simulink model "HT07CombinedPowertrainThermalModelv2IsolatedMotors"  (R2022b)
settings: Solver=VariableStepAuto  StartTime=0.0  StopTime=timeEnd  RelTol=1e-2
values from neighbouring files (symbols this model uses):
  radiator = dualPassRadiatorInit(radiator)    [HT07CombinedPowertrainThermalSetup.m]
  Tamb = 26    [HT07CombinedPowertrainThermalSetup.m]    (also in HT07PowertrainThermalSetup.m = 33; HT07PowertrainThermalSetupExperimental.m)
undefined symbols (not defined in the file or in its folder): AH, convectionArea, DiscIntNeverNeededParam, SOC0, startTempC, tabResis
libraries: fl_lib x165, nesl_utility x43, SimscapeFluids_lib x16, ee_lib x2
(part 2 of 5)

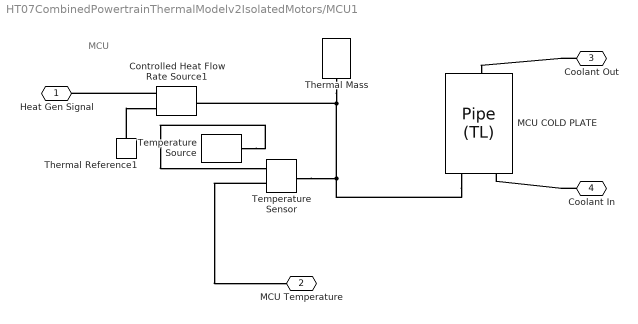
== system HT07CombinedPowertrainThermalModelv2IsolatedMotors/MCU1 ==
  note: MCU
  Controlled Heat Flow Rate Source1 : fl_lib/Thermal/Thermal Sources/Controlled Heat Flow Rate Source
  MCU COLD PLATE : SimscapeFluids_lib/Thermal Liquid/Pipes & Fittings/Pipe (TL)  dynamic_compressibility=simscape.enum.onoff.off  inertia=simscape.enum.onoff.off  num_segments=1  pipe_length=mcuColdPlateLength m  area=mcuColdPlateFlowArea m^2  wall_spec=fluids.thermal_liquid.pipes_fittings.enum.wall_spec.rigid  Dh=mcuColdPlateDiameter m  wall_compliance=1.2e-6 m/MPa  wall_time_constant=0.01 s  elevation_spec=foundation.enum.constant_variable.constant  elevation_gain=0 m  g=9.81 m/s^2  pressure_loss_spec=fluids.thermal_liquid.pipes_fittings.enum.PressureLossSpec.Nominal  local_pressure_loss_spec=fluids.thermal_liquid.pipes_fittings.enum.LocalLossSpec.AggregateLength  length_add=0 m  loss_coefficient=0.1  roughness=tubeRoughness m  Re_friction_TLU=[400, 1000, 1500, 3000, 4000, 6000, 10000, 20000, 40000, 60000, 100000, 100000000]  friction_factor_TLU=[.264, .112, .071, .0417, .0387, .0268, .025, .0232, .0226, .022, .0214, .0214]  shape_factor=64  Re_lam=2000  Re_tur=4000  mdot_nominal=12 kg/min  p_diff_nominal=0.3 bar  mdot_threshold=1e-6 kg/s  heat_transfer_spec=fluids.thermal_liquid.pipes_fittings.enum.HeatTransferSpec.DittusBoelter  mdot_nominal_heat=[.1, 1] kg/s  T_in_nominal=[293.15, 293.15] K  T_out_nominal=[300, 300] K  p_in_nominal_heat=[.101325, .101325] MPa  T_wall_nominal=[303.15, 303.15] K  a_coeff=0.023  b_Re_power=0.8  c_Pr_power=0.4  Nu_lam=3.66  Re_Colburn_TLU=[100, 150, 1000]  Colburn_factor_TLU=[.019, .013, .002]  Re_Nu_TLU=[100, 150, 1000]  Pr_Nu_TLU=[1, 10]  Nu_TLU=[3.72, 4.21; 3.75, 4.44; 4.21, 7.15]  T0_vec=Tamb degC  p0_vec=0.101325 MPa  mdot0=0.1 kg/s
  Temperature Sensor : fl_lib/Thermal/Thermal Sensors/Temperature Sensor
  Temperature Source : fl_lib/Thermal/Thermal Sources/Temperature Source  temperature=0 degC
  Thermal Mass : fl_lib/Thermal/Thermal Elements/Thermal Mass  mass=coldPlateMassMCU kg  sp_heat=cAl J/(K*kg)  num_ports=foundation.enum.numPorts2.one  T_specify=on  T_priority=High  T=Tamb degC  T_nominal_specify=off  T_nominal_unit=K  T_nominal_value=1  Q_specify=off  Q_priority=None  Q=0 W  Q_nominal_specify=off  Q_nominal_unit=W  Q_nominal_value=1
  Thermal Reference1 : fl_lib/Thermal/Thermal Elements/Thermal Reference
  Heat Gen Signal : PMIOPort  Side=Left
  MCU Temperature : PMIOPort  Port=2  Side=Left
  Coolant Out : PMIOPort  Port=3  Side=Right
  Coolant In : PMIOPort  Port=4  Side=Right
  connections:
  Temperature Sensor/RConn2 -- MCU Temperature/RConn1
  MCU COLD PLATE/LConn2 -- Temperature Sensor/LConn1 -- Thermal Mass/LConn1 -- Controlled Heat Flow Rate Source1/LConn1
  Temperature Source/LConn1 -- Temperature Sensor/RConn1
  Thermal Reference1/LConn1 -- Controlled Heat Flow Rate Source1/RConn2
  Coolant In/RConn1 -- MCU COLD PLATE/LConn1
  Coolant Out/RConn1 -- MCU COLD PLATE/RConn1
  Controlled Heat Flow Rate Source1/RConn1 -- Heat Gen Signal/RConn1

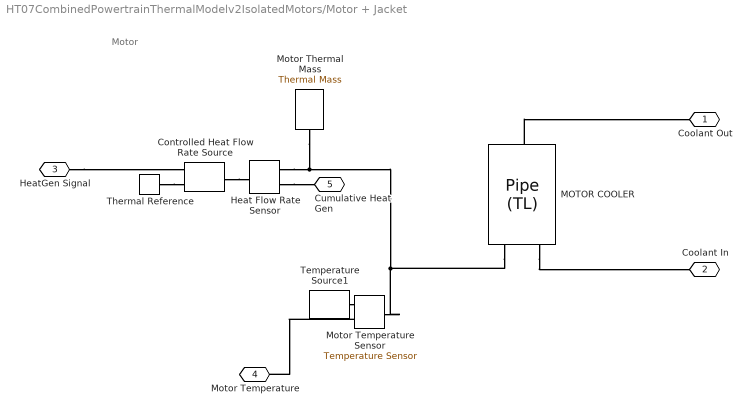
== system HT07CombinedPowertrainThermalModelv2IsolatedMotors/Motor + Jacket ==
  note: Motor
  Controlled Heat Flow Rate Source : fl_lib/Thermal/Thermal Sources/Controlled Heat Flow Rate Source
  Heat Flow Rate Sensor : fl_lib/Thermal/Thermal Sensors/Heat Flow Rate Sensor
  MOTOR COOLER : SimscapeFluids_lib/Thermal Liquid/Pipes & Fittings/Pipe (TL)  dynamic_compressibility=simscape.enum.onoff.off  inertia=simscape.enum.onoff.off  num_segments=1  pipe_length=motor.CoolingJacketLength m  area=motor.CoolingJacketFlowArea m^2  wall_spec=fluids.thermal_liquid.pipes_fittings.enum.wall_spec.rigid  Dh=motor.CoolingJacketHydraulicDiameter m  wall_compliance=1.2e-6 m/MPa  wall_time_constant=0.01 s  elevation_spec=foundation.enum.constant_variable.constant  elevation_gain=0 m  g=9.81 m/s^2  pressure_loss_spec=fluids.thermal_liquid.pipes_fittings.enum.PressureLossSpec.Haaland  local_pressure_loss_spec=fluids.thermal_liquid.pipes_fittings.enum.LocalLossSpec.AggregateLength  length_add=0 m  loss_coefficient=0.1  roughness=motor.CoolingJacketAbsoluteRoughness m  Re_friction_TLU=[400, 1000, 1500, 3000, 4000, 6000, 10000, 20000, 40000, 60000, 100000, 100000000]  friction_factor_TLU=[.264, .112, .071, .0417, .0387, .0268, .025, .0232, .0226, .022, .0214, .0214]  shape_factor=64  Re_lam=2000  Re_tur=4000  mdot_nominal=7 kg/min  p_diff_nominal=0.6 bar  mdot_threshold=1e-6 kg/s  heat_transfer_spec=fluids.thermal_liquid.pipes_fittings.enum.HeatTransferSpec.DittusBoelter  mdot_nominal_heat=[.1, 1] kg/s  T_in_nominal=[293.15, 293.15] K  T_out_nominal=[300, 300] K  p_in_nominal_heat=[.101325, .101325] MPa  T_wall_nominal=[303.15, 303.15] K  a_coeff=motor.DittusBoelterAadj  b_Re_power=0.8  c_Pr_power=0.4  Nu_lam=3.66  Re_Colburn_TLU=[100, 150, 1000]  Colburn_factor_TLU=[.019, .013, .002]  Re_Nu_TLU=[100, 150, 1000]  Pr_Nu_TLU=[1, 10]  Nu_TLU=[3.72, 4.21; 3.75, 4.44; 4.21, 7.15]  T0_vec=Tamb degC  p0_vec=0.101325 MPa  mdot0=0.1 kg/s
  Motor Temperature Sensor : fl_lib/Thermal/Thermal Sensors/Temperature Sensor
  Motor Thermal Mass : fl_lib/Thermal/Thermal Elements/Thermal Mass  mass=motor.Mass kg  sp_heat=cAl J/kg/K  num_ports=foundation.enum.numPorts2.one  T_specify=on  T_priority=High  T=Tamb degC  T_nominal_specify=off  T_nominal_unit=K  T_nominal_value=1  Q_specify=off  Q_priority=None  Q=0 W  Q_nominal_specify=off  Q_nominal_unit=W  Q_nominal_value=1
  Temperature Source1 : fl_lib/Thermal/Thermal Sources/Temperature Source  temperature=0 degC
  Thermal Reference : fl_lib/Thermal/Thermal Elements/Thermal Reference
  Coolant Out : PMIOPort  Side=Left
  Coolant In : PMIOPort  Port=2  Side=Left
  HeatGen Signal : PMIOPort  Port=3  Side=Right
  Motor Temperature : PMIOPort  Port=4  Side=Right
  Cumulative Heat Gen : PMIOPort  Port=5  Side=Right
  connections:
  Motor Thermal Mass/LConn1 -- Heat Flow Rate Sensor/RConn2 -- MOTOR COOLER/LConn2 -- Motor Temperature Sensor/LConn1
  Thermal Reference/LConn1 -- Controlled Heat Flow Rate Source/RConn2
  Temperature Source1/LConn1 -- Motor Temperature Sensor/RConn1
  Motor Temperature Sensor/RConn2 -- Motor Temperature/RConn1
  Controlled Heat Flow Rate Source/LConn1 -- Heat Flow Rate Sensor/LConn1
  MOTOR COOLER/RConn1 -- Coolant Out/RConn1
  MOTOR COOLER/LConn1 -- Coolant In/RConn1
  HeatGen Signal/RConn1 -- Controlled Heat Flow Rate Source/RConn1
  Heat Flow Rate Sensor/RConn1 -- Cumulative Heat Gen/RConn1

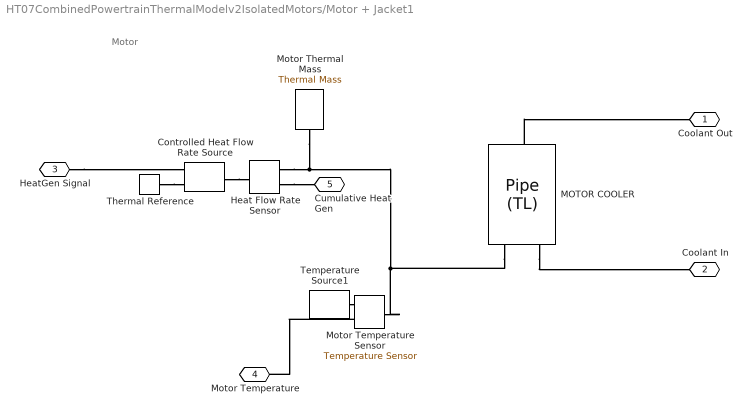
== system HT07CombinedPowertrainThermalModelv2IsolatedMotors/Motor + Jacket1 ==
  note: Motor
  Controlled Heat Flow Rate Source : fl_lib/Thermal/Thermal Sources/Controlled Heat Flow Rate Source
  Heat Flow Rate Sensor : fl_lib/Thermal/Thermal Sensors/Heat Flow Rate Sensor
  MOTOR COOLER : SimscapeFluids_lib/Thermal Liquid/Pipes & Fittings/Pipe (TL)  dynamic_compressibility=simscape.enum.onoff.off  inertia=simscape.enum.onoff.off  num_segments=1  pipe_length=motor.CoolingJacketLength m  area=motor.CoolingJacketFlowArea m^2  wall_spec=fluids.thermal_liquid.pipes_fittings.enum.wall_spec.rigid  Dh=motor.CoolingJacketHydraulicDiameter m  wall_compliance=1.2e-6 m/MPa  wall_time_constant=0.01 s  elevation_spec=foundation.enum.constant_variable.constant  elevation_gain=0 m  g=9.81 m/s^2  pressure_loss_spec=fluids.thermal_liquid.pipes_fittings.enum.PressureLossSpec.Haaland  local_pressure_loss_spec=fluids.thermal_liquid.pipes_fittings.enum.LocalLossSpec.AggregateLength  length_add=0 m  loss_coefficient=0.1  roughness=motor.CoolingJacketAbsoluteRoughness m  Re_friction_TLU=[400, 1000, 1500, 3000, 4000, 6000, 10000, 20000, 40000, 60000, 100000, 100000000]  friction_factor_TLU=[.264, .112, .071, .0417, .0387, .0268, .025, .0232, .0226, .022, .0214, .0214]  shape_factor=64  Re_lam=2000  Re_tur=4000  mdot_nominal=7 kg/min  p_diff_nominal=0.6 bar  mdot_threshold=1e-6 kg/s  heat_transfer_spec=fluids.thermal_liquid.pipes_fittings.enum.HeatTransferSpec.DittusBoelter  mdot_nominal_heat=[.1, 1] kg/s  T_in_nominal=[293.15, 293.15] K  T_out_nominal=[300, 300] K  p_in_nominal_heat=[.101325, .101325] MPa  T_wall_nominal=[303.15, 303.15] K  a_coeff=motor.DittusBoelterAadj  b_Re_power=0.8  c_Pr_power=0.4  Nu_lam=3.66  Re_Colburn_TLU=[100, 150, 1000]  Colburn_factor_TLU=[.019, .013, .002]  Re_Nu_TLU=[100, 150, 1000]  Pr_Nu_TLU=[1, 10]  Nu_TLU=[3.72, 4.21; 3.75, 4.44; 4.21, 7.15]  T0_vec=Tamb degC  p0_vec=0.101325 MPa  mdot0=0.1 kg/s
  Motor Temperature Sensor : fl_lib/Thermal/Thermal Sensors/Temperature Sensor
  Motor Thermal Mass : fl_lib/Thermal/Thermal Elements/Thermal Mass  mass=motor.Mass kg  sp_heat=cAl J/kg/K  num_ports=foundation.enum.numPorts2.one  T_specify=on  T_priority=High  T=Tamb degC  T_nominal_specify=off  T_nominal_unit=K  T_nominal_value=1  Q_specify=off  Q_priority=None  Q=0 W  Q_nominal_specify=off  Q_nominal_unit=W  Q_nominal_value=1
  Temperature Source1 : fl_lib/Thermal/Thermal Sources/Temperature Source  temperature=0 degC
  Thermal Reference : fl_lib/Thermal/Thermal Elements/Thermal Reference
  Coolant Out : PMIOPort  Side=Left
  Coolant In : PMIOPort  Port=2  Side=Left
  HeatGen Signal : PMIOPort  Port=3  Side=Right
  Motor Temperature : PMIOPort  Port=4  Side=Right
  Cumulative Heat Gen : PMIOPort  Port=5  Side=Right
  connections:
  Motor Temperature Sensor/LConn1 -- MOTOR COOLER/LConn2 -- Motor Thermal Mass/LConn1 -- Heat Flow Rate Sensor/RConn2
  Thermal Reference/LConn1 -- Controlled Heat Flow Rate Source/RConn2
  Temperature Source1/LConn1 -- Motor Temperature Sensor/RConn1
  Motor Temperature Sensor/RConn2 -- Motor Temperature/RConn1
  Controlled Heat Flow Rate Source/LConn1 -- Heat Flow Rate Sensor/LConn1
  MOTOR COOLER/RConn1 -- Coolant Out/RConn1
  MOTOR COOLER/LConn1 -- Coolant In/RConn1
  HeatGen Signal/RConn1 -- Controlled Heat Flow Rate Source/RConn1
  Heat Flow Rate Sensor/RConn1 -- Cumulative Heat Gen/RConn1

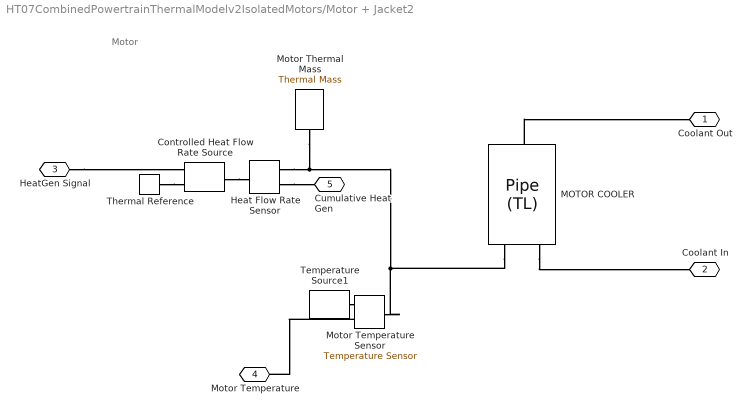
== system HT07CombinedPowertrainThermalModelv2IsolatedMotors/Motor + Jacket2 ==
  note: Motor
  Controlled Heat Flow Rate Source : fl_lib/Thermal/Thermal Sources/Controlled Heat Flow Rate Source
  Heat Flow Rate Sensor : fl_lib/Thermal/Thermal Sensors/Heat Flow Rate Sensor
  MOTOR COOLER : SimscapeFluids_lib/Thermal Liquid/Pipes & Fittings/Pipe (TL)  dynamic_compressibility=simscape.enum.onoff.off  inertia=simscape.enum.onoff.off  num_segments=1  pipe_length=motor.CoolingJacketLength m  area=motor.CoolingJacketFlowArea m^2  wall_spec=fluids.thermal_liquid.pipes_fittings.enum.wall_spec.rigid  Dh=motor.CoolingJacketHydraulicDiameter m  wall_compliance=1.2e-6 m/MPa  wall_time_constant=0.01 s  elevation_spec=foundation.enum.constant_variable.constant  elevation_gain=0 m  g=9.81 m/s^2  pressure_loss_spec=fluids.thermal_liquid.pipes_fittings.enum.PressureLossSpec.Haaland  local_pressure_loss_spec=fluids.thermal_liquid.pipes_fittings.enum.LocalLossSpec.AggregateLength  length_add=0 m  loss_coefficient=0.1  roughness=motor.CoolingJacketAbsoluteRoughness m  Re_friction_TLU=[400, 1000, 1500, 3000, 4000, 6000, 10000, 20000, 40000, 60000, 100000, 100000000]  friction_factor_TLU=[.264, .112, .071, .0417, .0387, .0268, .025, .0232, .0226, .022, .0214, .0214]  shape_factor=64  Re_lam=2000  Re_tur=4000  mdot_nominal=7 kg/min  p_diff_nominal=0.6 bar  mdot_threshold=1e-6 kg/s  heat_transfer_spec=fluids.thermal_liquid.pipes_fittings.enum.HeatTransferSpec.DittusBoelter  mdot_nominal_heat=[.1, 1] kg/s  T_in_nominal=[293.15, 293.15] K  T_out_nominal=[300, 300] K  p_in_nominal_heat=[.101325, .101325] MPa  T_wall_nominal=[303.15, 303.15] K  a_coeff=motor.DittusBoelterAadj  b_Re_power=0.8  c_Pr_power=0.4  Nu_lam=3.66  Re_Colburn_TLU=[100, 150, 1000]  Colburn_factor_TLU=[.019, .013, .002]  Re_Nu_TLU=[100, 150, 1000]  Pr_Nu_TLU=[1, 10]  Nu_TLU=[3.72, 4.21; 3.75, 4.44; 4.21, 7.15]  T0_vec=Tamb degC  p0_vec=0.101325 MPa  mdot0=0.1 kg/s
  Motor Temperature Sensor : fl_lib/Thermal/Thermal Sensors/Temperature Sensor
  Motor Thermal Mass : fl_lib/Thermal/Thermal Elements/Thermal Mass  mass=motor.Mass kg  sp_heat=cAl J/kg/K  num_ports=foundation.enum.numPorts2.one  T_specify=on  T_priority=High  T=Tamb degC  T_nominal_specify=off  T_nominal_unit=K  T_nominal_value=1  Q_specify=off  Q_priority=None  Q=0 W  Q_nominal_specify=off  Q_nominal_unit=W  Q_nominal_value=1
  Temperature Source1 : fl_lib/Thermal/Thermal Sources/Temperature Source  temperature=0 degC
  Thermal Reference : fl_lib/Thermal/Thermal Elements/Thermal Reference
  Coolant Out : PMIOPort  Side=Left
  Coolant In : PMIOPort  Port=2  Side=Left
  HeatGen Signal : PMIOPort  Port=3  Side=Right
  Motor Temperature : PMIOPort  Port=4  Side=Right
  Cumulative Heat Gen : PMIOPort  Port=5  Side=Right
  connections:
  Motor Temperature Sensor/LConn1 -- MOTOR COOLER/LConn2 -- Motor Thermal Mass/LConn1 -- Heat Flow Rate Sensor/RConn2
  Thermal Reference/LConn1 -- Controlled Heat Flow Rate Source/RConn2
  Temperature Source1/LConn1 -- Motor Temperature Sensor/RConn1
  Motor Temperature Sensor/RConn2 -- Motor Temperature/RConn1
  Controlled Heat Flow Rate Source/LConn1 -- Heat Flow Rate Sensor/LConn1
  MOTOR COOLER/RConn1 -- Coolant Out/RConn1
  MOTOR COOLER/LConn1 -- Coolant In/RConn1
  HeatGen Signal/RConn1 -- Controlled Heat Flow Rate Source/RConn1
  Heat Flow Rate Sensor/RConn1 -- Cumulative Heat Gen/RConn1

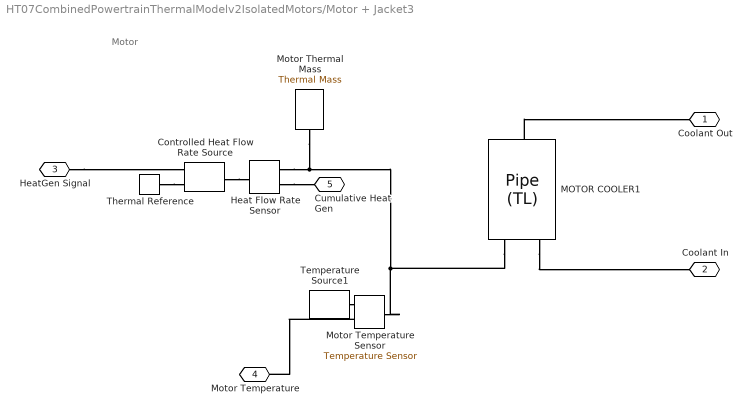
== system HT07CombinedPowertrainThermalModelv2IsolatedMotors/Motor + Jacket3 ==
  note: Motor
  Controlled Heat Flow Rate Source : fl_lib/Thermal/Thermal Sources/Controlled Heat Flow Rate Source
  Heat Flow Rate Sensor : fl_lib/Thermal/Thermal Sensors/Heat Flow Rate Sensor
  MOTOR COOLER1 : SimscapeFluids_lib/Thermal Liquid/Pipes & Fittings/Pipe (TL)  dynamic_compressibility=simscape.enum.onoff.off  inertia=simscape.enum.onoff.off  num_segments=1  pipe_length=motor.CoolingJacketLength m  area=motor.CoolingJacketFlowArea m^2  wall_spec=fluids.thermal_liquid.pipes_fittings.enum.wall_spec.rigid  Dh=motor.CoolingJacketHydraulicDiameter m  wall_compliance=1.2e-6 m/MPa  wall_time_constant=0.01 s  elevation_spec=foundation.enum.constant_variable.constant  elevation_gain=0 m  g=9.81 m/s^2  pressure_loss_spec=fluids.thermal_liquid.pipes_fittings.enum.PressureLossSpec.Haaland  local_pressure_loss_spec=fluids.thermal_liquid.pipes_fittings.enum.LocalLossSpec.AggregateLength  length_add=0 m  loss_coefficient=0.1  roughness=motor.CoolingJacketAbsoluteRoughness m  Re_friction_TLU=[400, 1000, 1500, 3000, 4000, 6000, 10000, 20000, 40000, 60000, 100000, 100000000]  friction_factor_TLU=[.264, .112, .071, .0417, .0387, .0268, .025, .0232, .0226, .022, .0214, .0214]  shape_factor=64  Re_lam=2000  Re_tur=4000  mdot_nominal=7 kg/min  p_diff_nominal=0.6 bar  mdot_threshold=1e-6 kg/s  heat_transfer_spec=fluids.thermal_liquid.pipes_fittings.enum.HeatTransferSpec.DittusBoelter  mdot_nominal_heat=[.1, 1] kg/s  T_in_nominal=[293.15, 293.15] K  T_out_nominal=[300, 300] K  p_in_nominal_heat=[.101325, .101325] MPa  T_wall_nominal=[303.15, 303.15] K  a_coeff=motor.DittusBoelterAadj  b_Re_power=0.8  c_Pr_power=0.4  Nu_lam=3.66  Re_Colburn_TLU=[100, 150, 1000]  Colburn_factor_TLU=[.019, .013, .002]  Re_Nu_TLU=[100, 150, 1000]  Pr_Nu_TLU=[1, 10]  Nu_TLU=[3.72, 4.21; 3.75, 4.44; 4.21, 7.15]  T0_vec=Tamb degC  p0_vec=0.101325 MPa  mdot0=0.1 kg/s
  Motor Temperature Sensor : fl_lib/Thermal/Thermal Sensors/Temperature Sensor
  Motor Thermal Mass : fl_lib/Thermal/Thermal Elements/Thermal Mass  mass=motor.Mass kg  sp_heat=cAl J/kg/K  num_ports=foundation.enum.numPorts2.one  T_specify=on  T_priority=High  T=Tamb degC  T_nominal_specify=off  T_nominal_unit=K  T_nominal_value=1  Q_specify=off  Q_priority=None  Q=0 W  Q_nominal_specify=off  Q_nominal_unit=W  Q_nominal_value=1
  Temperature Source1 : fl_lib/Thermal/Thermal Sources/Temperature Source  temperature=0 degC
  Thermal Reference : fl_lib/Thermal/Thermal Elements/Thermal Reference
  Coolant Out : PMIOPort  Side=Left
  Coolant In : PMIOPort  Port=2  Side=Left
  HeatGen Signal : PMIOPort  Port=3  Side=Right
  Motor Temperature : PMIOPort  Port=4  Side=Right
  Cumulative Heat Gen : PMIOPort  Port=5  Side=Right
  connections:
  Motor Temperature Sensor/LConn1 -- MOTOR COOLER1/LConn2 -- Motor Thermal Mass/LConn1 -- Heat Flow Rate Sensor/RConn2
  Thermal Reference/LConn1 -- Controlled Heat Flow Rate Source/RConn2
  Temperature Source1/LConn1 -- Motor Temperature Sensor/RConn1
  Motor Temperature Sensor/RConn2 -- Motor Temperature/RConn1
  Controlled Heat Flow Rate Source/LConn1 -- Heat Flow Rate Sensor/LConn1
  MOTOR COOLER1/RConn1 -- Coolant Out/RConn1
  MOTOR COOLER1/LConn1 -- Coolant In/RConn1
  HeatGen Signal/RConn1 -- Controlled Heat Flow Rate Source/RConn1
  Heat Flow Rate Sensor/RConn1 -- Cumulative Heat Gen/RConn1

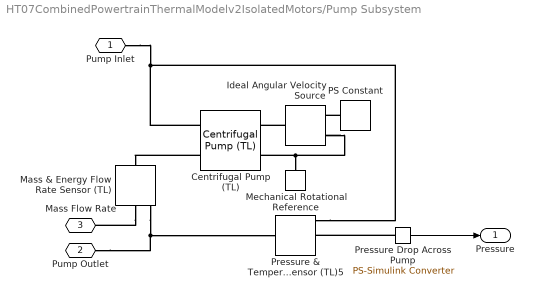
== system HT07CombinedPowertrainThermalModelv2IsolatedMotors/Pump Subsystem ==
  Centrifugal Pump (TL) : SimscapeFluids_lib/Thermal Liquid/Pumps & Motors/Centrifugal Pump (TL)  pump_parameterization=fluids.thermal_liquid.pumps_motors.enum.CentrifugalPumpParameterization.Table1D  capacity_ref_nominal=45 lpm  head_ref_nominal=40 m  power_ref_nominal=0.85 kW  head_ref_max=60 m  capacity_ref_max=80 lpm  omega_ref_analytic=1770 rpm  flow_rate_1D_TLU=pumpCapacity lpm  head_1D_TLU=pumpHead m  power_1D_TLU=pumpPower W  omega_ref_1D=3500 rpm  rho_ref_1D=998.21 kg/m^3  flow_rate_2D_TLU=[16.67, 23.33, 30, 40, 53.33, 60] lpm  omega_2D_TLU=[2450, 2800, 3150, 3500] rpm  head_2D_TLU=[25, 32.7, 42.5, 50; 24, 31.7, 41, 49; 22.7, 30.5, 39, 47.5; 20, 28, 36, 45; 15.7, 24, 32, 40; 12.5, 21, 29.5, 37.5] m  power_2D_TLU=[.28, .38, .5, .6; .31, .41, .55, .68; .33, .44, .6, .75; .36, .48, .65, .83; .38, .53, .72, .93; .39, .55, .75, .97] kW  rho_ref_2D=998.21 kg/m^3  diameter_ratio=1  mech_orientation=fluids.thermal_liquid.pumps_motors.enum.CentrifugalPumpMechOrientation.Positive  area=0.019 ^ 2 / 4 *pi m^2
      settings: InternalSimscapePortConfiguration="{\"Bottom\":[],\"Left\":[{\"id\":\"A\",\"label\":\"A\",\"type\":\"foundation.thermal_liquid.thermal_liquid\"},{\"id\":\"B\",\"label\":\"B\",\"type\":\"foundation.thermal_liquid.thermal_liquid\"}],\"Right\":[{\"id\":\"R\",\"label\":\"R\",\"type\":\"foundation.mechanical.rotational.rotational\"},{\"id\":\"C\",\"label\":\"C\",\"type\":\"foundation.mechanical.rotational.rotational\"}],\"Top\":[]}"
  Ideal Angular Velocity Source : fl_lib/Mechanical/Mechanical Sources/Ideal Angular Velocity Source
  Mass & Energy Flow Rate Sensor (TL) : fl_lib/Thermal Liquid/Sensors/Mass & Energy Flow Rate Sensor (TL)
      settings: InternalSimscapePortConfiguration="{\"Bottom\":[],\"Left\":[{\"id\":\"A\",\"label\":\"A\",\"type\":\"foundation.thermal_liquid.thermal_liquid\"}],\"Right\":[{\"id\":\"B\",\"label\":\"B\",\"type\":\"foundation.thermal_liquid.thermal_liquid\"},{\"id\":\"M\",\"label\":\"M\",\"type\":\"output\"},{\"id\":\"PHI\",\"label\":\"Phi\",\"type\":\"output\"}],\"Top\":[]}"
  Mechanical Rotational Reference : fl_lib/Mechanical/Rotational Elements/Mechanical Rotational Reference
  PS Constant : fl_lib/Physical Signals/Sources/PS Constant  constant=3500 rpm
  Pressure & Temperature Sensor (TL)5 : fl_lib/Thermal Liquid/Sensors/Pressure & Temperature Sensor (TL)
      settings: InternalSimscapePortConfiguration="{\"Bottom\":[],\"Left\":[{\"id\":\"A\",\"label\":\"A\",\"type\":\"foundation.thermal_liquid.thermal_liquid\"}],\"Right\":[{\"id\":\"B\",\"label\":\"B\",\"type\":\"foundation.thermal_liquid.thermal_liquid\"},{\"id\":\"P\",\"label\":\"P\",\"type\":\"output\"},{\"id\":\"T\",\"label\":\"T\",\"type\":\"output\"}],\"Top\":[]}"
  Pressure Drop Across Pump : nesl_utility/PS-Simulink Converter  PhysicalDomain=network_engine_domain  SubClassName=ps_output  LeftPortType=input  RightPortType=output  PseudoPeriodic=off  Frequencies=[]  VectorFormat=1-D array  Unit=inherit  AffineConversion=off
  Pump Inlet : PMIOPort  Side=Left
  Pump Outlet : PMIOPort  Port=2  Side=Left
  Mass Flow Rate : PMIOPort  Port=3  Side=Right
  Pressure : Outport
  wires:
  Pressure Drop Across Pump/1 -> Pressure/1
  connections:
  Pressure & Temperature Sensor (TL)5/RConn1 -- Pump Inlet/RConn1 -- Centrifugal Pump (TL)/LConn1
  Pump Outlet/RConn1 -- Pressure & Temperature Sensor (TL)5/LConn1 -- Mass & Energy Flow Rate Sensor (TL)/RConn1
  Ideal Angular Velocity Source/RConn2 -- Centrifugal Pump (TL)/RConn2 -- Mechanical Rotational Reference/LConn1
  PS Constant/RConn1 -- Ideal Angular Velocity Source/RConn1
  Ideal Angular Velocity Source/LConn1 -- Centrifugal Pump (TL)/RConn1
  Pressure Drop Across Pump/LConn1 -- Pressure & Temperature Sensor (TL)5/RConn2
  Mass & Energy Flow Rate Sensor (TL)/RConn2 -- Mass Flow Rate/RConn1
  Centrifugal Pump (TL)/LConn2 -- Mass & Energy Flow Rate Sensor (TL)/LConn1

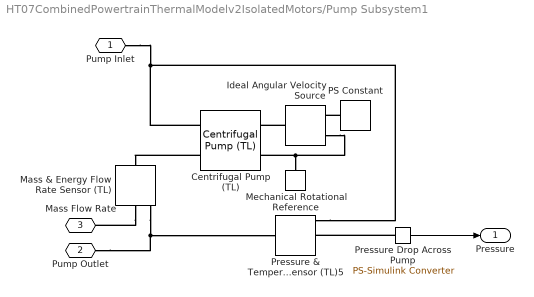
== system HT07CombinedPowertrainThermalModelv2IsolatedMotors/Pump Subsystem1 ==
  Centrifugal Pump (TL) : SimscapeFluids_lib/Thermal Liquid/Pumps & Motors/Centrifugal Pump (TL)  pump_parameterization=fluids.thermal_liquid.pumps_motors.enum.CentrifugalPumpParameterization.Table1D  capacity_ref_nominal=45 lpm  head_ref_nominal=40 m  power_ref_nominal=0.85 kW  head_ref_max=60 m  capacity_ref_max=80 lpm  omega_ref_analytic=1770 rpm  flow_rate_1D_TLU=pumpCapacity lpm  head_1D_TLU=pumpHead m  power_1D_TLU=pumpPower W  omega_ref_1D=3500 rpm  rho_ref_1D=998.21 kg/m^3  flow_rate_2D_TLU=[16.67, 23.33, 30, 40, 53.33, 60] lpm  omega_2D_TLU=[2450, 2800, 3150, 3500] rpm  head_2D_TLU=[25, 32.7, 42.5, 50; 24, 31.7, 41, 49; 22.7, 30.5, 39, 47.5; 20, 28, 36, 45; 15.7, 24, 32, 40; 12.5, 21, 29.5, 37.5] m  power_2D_TLU=[.28, .38, .5, .6; .31, .41, .55, .68; .33, .44, .6, .75; .36, .48, .65, .83; .38, .53, .72, .93; .39, .55, .75, .97] kW  rho_ref_2D=998.21 kg/m^3  diameter_ratio=1  mech_orientation=fluids.thermal_liquid.pumps_motors.enum.CentrifugalPumpMechOrientation.Positive  area=0.019 ^ 2 / 4 *pi m^2
      settings: InternalSimscapePortConfiguration="{\"Bottom\":[],\"Left\":[{\"id\":\"A\",\"label\":\"A\",\"type\":\"foundation.thermal_liquid.thermal_liquid\"},{\"id\":\"B\",\"label\":\"B\",\"type\":\"foundation.thermal_liquid.thermal_liquid\"}],\"Right\":[{\"id\":\"R\",\"label\":\"R\",\"type\":\"foundation.mechanical.rotational.rotational\"},{\"id\":\"C\",\"label\":\"C\",\"type\":\"foundation.mechanical.rotational.rotational\"}],\"Top\":[]}"
  Ideal Angular Velocity Source : fl_lib/Mechanical/Mechanical Sources/Ideal Angular Velocity Source
  Mass & Energy Flow Rate Sensor (TL) : fl_lib/Thermal Liquid/Sensors/Mass & Energy Flow Rate Sensor (TL)
      settings: InternalSimscapePortConfiguration="{\"Bottom\":[],\"Left\":[{\"id\":\"A\",\"label\":\"A\",\"type\":\"foundation.thermal_liquid.thermal_liquid\"}],\"Right\":[{\"id\":\"B\",\"label\":\"B\",\"type\":\"foundation.thermal_liquid.thermal_liquid\"},{\"id\":\"M\",\"label\":\"M\",\"type\":\"output\"},{\"id\":\"PHI\",\"label\":\"Phi\",\"type\":\"output\"}],\"Top\":[]}"
  Mechanical Rotational Reference : fl_lib/Mechanical/Rotational Elements/Mechanical Rotational Reference
  PS Constant : fl_lib/Physical Signals/Sources/PS Constant  constant=3500 rpm
  Pressure & Temperature Sensor (TL)5 : fl_lib/Thermal Liquid/Sensors/Pressure & Temperature Sensor (TL)
      settings: InternalSimscapePortConfiguration="{\"Bottom\":[],\"Left\":[{\"id\":\"A\",\"label\":\"A\",\"type\":\"foundation.thermal_liquid.thermal_liquid\"}],\"Right\":[{\"id\":\"B\",\"label\":\"B\",\"type\":\"foundation.thermal_liquid.thermal_liquid\"},{\"id\":\"P\",\"label\":\"P\",\"type\":\"output\"},{\"id\":\"T\",\"label\":\"T\",\"type\":\"output\"}],\"Top\":[]}"
  Pressure Drop Across Pump : nesl_utility/PS-Simulink Converter  PhysicalDomain=network_engine_domain  SubClassName=ps_output  LeftPortType=input  RightPortType=output  PseudoPeriodic=off  Frequencies=[]  VectorFormat=1-D array  Unit=inherit  AffineConversion=off
  Pump Inlet : PMIOPort  Side=Left
  Pump Outlet : PMIOPort  Port=2  Side=Left
  Mass Flow Rate : PMIOPort  Port=3  Side=Right
  Pressure : Outport
  wires:
  Pressure Drop Across Pump/1 -> Pressure/1
  connections:
  Pressure & Temperature Sensor (TL)5/RConn1 -- Centrifugal Pump (TL)/LConn1 -- Pump Inlet/RConn1
  Pump Outlet/RConn1 -- Mass & Energy Flow Rate Sensor (TL)/RConn1 -- Pressure & Temperature Sensor (TL)5/LConn1
  Ideal Angular Velocity Source/RConn2 -- Centrifugal Pump (TL)/RConn2 -- Mechanical Rotational Reference/LConn1
  PS Constant/RConn1 -- Ideal Angular Velocity Source/RConn1
  Ideal Angular Velocity Source/LConn1 -- Centrifugal Pump (TL)/RConn1
  Pressure Drop Across Pump/LConn1 -- Pressure & Temperature Sensor (TL)5/RConn2
  Mass & Energy Flow Rate Sensor (TL)/RConn2 -- Mass Flow Rate/RConn1
  Centrifugal Pump (TL)/LConn2 -- Mass & Energy Flow Rate Sensor (TL)/LConn1
